simulink model "ExtendedKalmanFIlterRover"  (R2021a)
settings: Solver=VariableStepAuto  StartTime=0.0  StopTime=20.0  RelTol=1e-3
values from neighbouring files (symbols this model uses):
  Q = 1.2e-3    (= 0.0012)    [parameters.m]
  R = 5e-3    (= 0.005)    [parameters.m]
  Ts = 0.01    [parameters.m]
undefined symbols (not defined in the file or in its folder): K
libraries: robotlib x9, sharedTrackingLibrary x1
settings Model: Creator=user  LastModifiedBy=User
settings SolverCC: AlgebraicLoopSolver=TrustRegion
settings DebuggingCC: SFMachineParentedDataDiag=warning

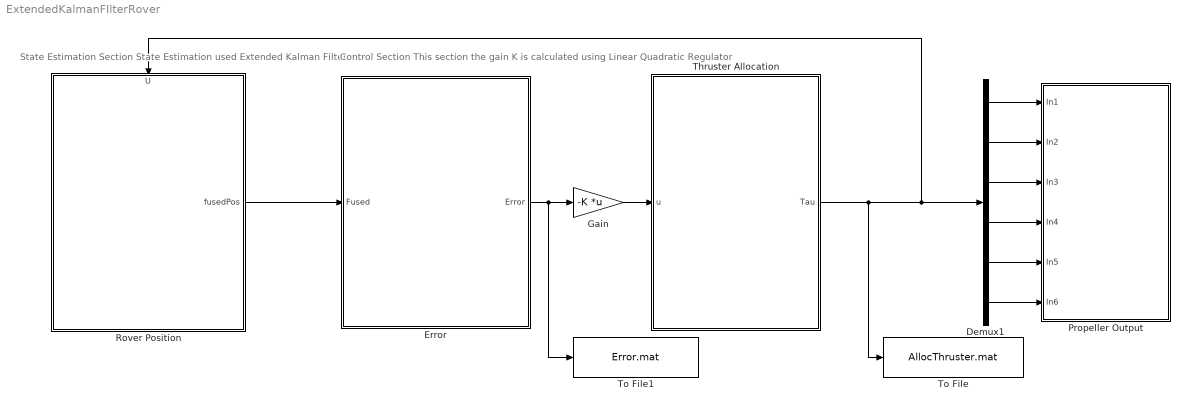
== system ExtendedKalmanFIlterRover ==
  note: State Estimation Section
      |
      | State Estimation used Extended Kalman Filter
  note: Control Section
      |
      | This section the gain K is calculated using Linear Quadratic Regulator
  Demux1 : Demux  Outputs=6
  Error : MATLAB Function  TreatAsAtomicUnit=on
  Gain : Gain  Gain=-K  Multiplication=Matrix(K*u)  RndMeth=Round
  Propeller Output : Subsystem
  Rover Position : Subsystem
      settings: PortSchema="{\"entries\":[{\"content\":{\"sides\":[{\"content\":{\"connectorIds\":[]},\"type\":\"ConnectorPlacement.EquallySpacedRectSide\",\"uuid\":\"70bf1008-d6b2-49b6-af88-753ab581769c\"},{\"content\":{\"connectorIds\":[\"Out1\"],\"side\":\"RIGHT\"},\"type\":\"ConnectorPlacement.EquallySpacedRectSide\",\"uuid\":\"04ddecda-8c46-4437-987b-fe54c22cd984\"},{\"content\":{\"connectorIds\":[\"In1\"],\"side\":\"TOP\"},\"type\":\"ConnectorPlacement.EquallySpacedRectSide\",\"uuid\":\"625a0b2a-12f2-4858-86ad-539843868268\"}]},\"type\":\"ConnectorPlacement.EquallySpacedConnector\",\"uuid\":\"e8b3dc5a-c0d9-4ca2-a6c5-b2c7be1821de\"}],\"packageUris\":[\"http://schema.mathworks.com/mf0/Connector/R2020b\"],\"version\":\"1.0\"}"
  Thruster Allocation : MATLAB Function  TreatAsAtomicUnit=on
  To File : ToFile  Filename=AllocThruster.mat  SaveFormat=Timeseries  SampleTime=Ts
  To File1 : ToFile  Filename=Error.mat  MatrixName=Error  SaveFormat=Timeseries  SampleTime=Ts
  wires:
  Thruster Allocation/1(Tau) -> To File/1, Demux1/1, Rover Position/1(U)
  Demux1/1 -> Propeller Output/1(In1)
  Demux1/2 -> Propeller Output/2(In2)
  Demux1/3 -> Propeller Output/3(In3)
  Demux1/4 -> Propeller Output/4(In4)
  Demux1/5 -> Propeller Output/5(In5)
  Demux1/6 -> Propeller Output/6(In6)
  Error/1(Error) -> To File1/1, Gain/1
  Rover Position/1(fusedPos) -> Error/1(Fused)
  Gain/1 -> Thruster Allocation/1(u)

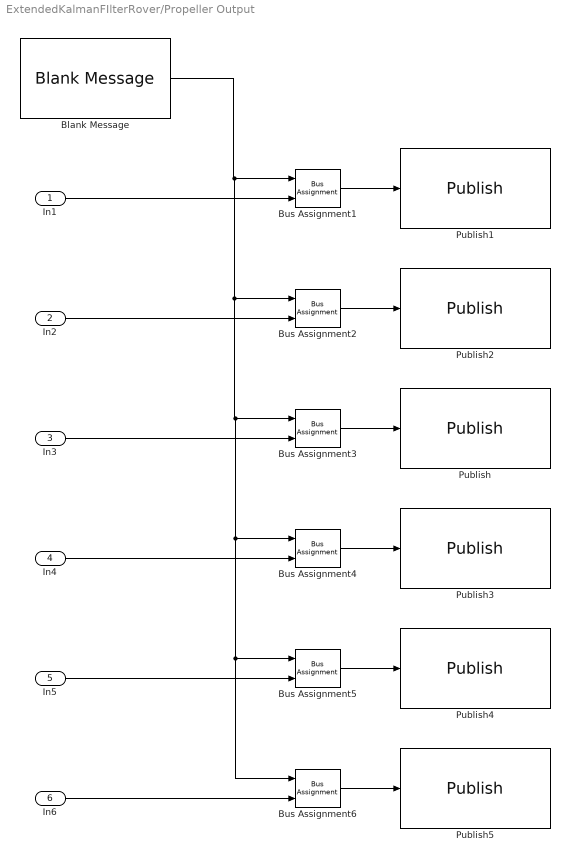
== system ExtendedKalmanFIlterRover/Propeller Output ==
  In1 : Inport
  In2 : Inport  Port=2
  In3 : Inport  Port=3
  In4 : Inport  Port=4
  In5 : Inport  Port=5
  In6 : Inport  Port=6
  Blank Message : robotlib/Blank Message  messageClass=Message  entityType=uuv_gazebo_ros_plugins_msgs/FloatStamped  messageType=uuv_gazebo_ros_plugins_msgs/FloatStamped  SampleTime=inf  legacyBusStruct=off
  Bus Assignment{1..6} (6 alike) : BusAssignment  AssignedSignals=Data
  Publish : robotlib/Publish  topicSource=Select from ROS network  topic=/bluerov2/thrusters/2/input  messageType=uuv_gazebo_ros_plugins_msgs/FloatStamped  legacyBusStruct=off  messageQueueLength=1
  Publish1 : robotlib/Publish  topicSource=Select from ROS network  topic=/bluerov2/thrusters/0/input  messageType=uuv_gazebo_ros_plugins_msgs/FloatStamped  legacyBusStruct=off  messageQueueLength=1
  Publish2 : robotlib/Publish  topicSource=Select from ROS network  topic=/bluerov2/thrusters/1/input  messageType=uuv_gazebo_ros_plugins_msgs/FloatStamped  legacyBusStruct=off  messageQueueLength=1
  Publish3 : robotlib/Publish  topicSource=Select from ROS network  topic=/bluerov2/thrusters/3/input  messageType=uuv_gazebo_ros_plugins_msgs/FloatStamped  legacyBusStruct=off  messageQueueLength=1
  Publish4 : robotlib/Publish  topicSource=Select from ROS network  topic=/bluerov2/thrusters/4/input  messageType=uuv_gazebo_ros_plugins_msgs/FloatStamped  legacyBusStruct=off  messageQueueLength=1
  Publish5 : robotlib/Publish  topicSource=Select from ROS network  topic=/bluerov2/thrusters/5/input  messageType=uuv_gazebo_ros_plugins_msgs/FloatStamped  legacyBusStruct=off  messageQueueLength=1
  wires:
  Bus Assignment5/1 -> Publish4/1
  Bus Assignment4/1 -> Publish3/1
  Bus Assignment3/1 -> Publish/1
  Bus Assignment2/1 -> Publish2/1
  Bus Assignment1/1 -> Publish1/1
  Bus Assignment6/1 -> Publish5/1
  Blank Message/1 -> Bus Assignment6/1, Bus Assignment5/1, Bus Assignment4/1, Bus Assignment3/1, Bus Assignment2/1, Bus Assignment1/1
  In1/1 -> Bus Assignment1/2
  In2/1 -> Bus Assignment2/2
  In3/1 -> Bus Assignment3/2
  In4/1 -> Bus Assignment4/2
  In5/1 -> Bus Assignment5/2
  In6/1 -> Bus Assignment6/2

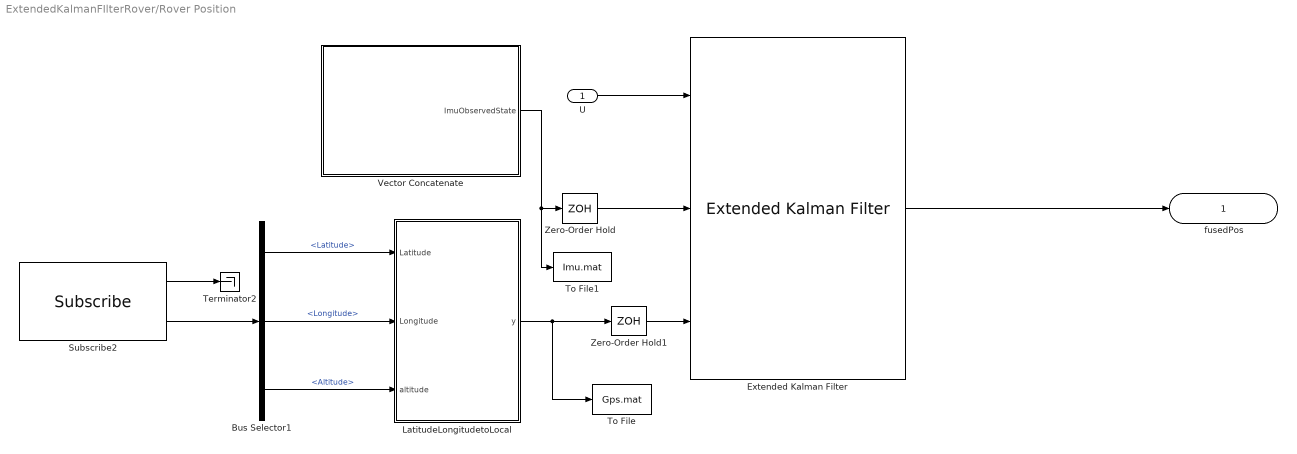
== system ExtendedKalmanFIlterRover/Rover Position ==
  U : Inport
  Bus Selector1 : BusSelector  OutputSignals=Latitude,Longitude,Altitude
  Extended Kalman Filter : sharedTrackingLibrary/Extended Kalman Filter  StateTransitionFcn=myStateTransitionFcn  HasStateTransitionJacobianFcn=off  HasAdditiveProcessNoise=Additive  ProcessNoise=diag([Q Q Q Q Q Q Q Q Q Q Q Q])  HasTimeVaryingProcessNoise=off  HasStateTransitionFcnExtraArgument=1  InitialState=[0 0 0 0 0 0 0 0 0 0 0 0]  InitialStateCovariance=1e-3  MeasurementFcn1=ImuMeasurementFcn  HasMeasurementJacobianFcn1=off  HasMeasurementEnablePort1=off  HasAdditiveMeasurementNoise1=Additive  MeasurementNoise1=diag([R R R R R R R R R R R R])  HasTimeVaryingMeasurementNoise1=off  HasMeasurementFcnExtraArgument1=0  MeasurementFcn2=GpsMeasurementFcn  HasMeasurementJacobianFcn2=off  HasMeasurementEnablePort2=off  HasAdditiveMeasurementNoise2=Additive  MeasurementNoise2=diag([R R R])  HasTimeVaryingMeasurementNoise2=off  HasMeasurementFcnExtraArgument2=0  MeasurementFcn3=myMeasurementFcn  HasMeasurementJacobianFcn3=off  HasMeasurementEnablePort3=off  HasAdditiveMeasurementNoise3=Additive  MeasurementNoise3=1  HasTimeVaryingMeasurementNoise3=off  HasMeasurementFcnExtraArgument3=0  MeasurementFcn4=myMeasurementFcn  HasMeasurementJacobianFcn4=off  HasMeasurementEnablePort4=off  HasAdditiveMeasurementNoise4=Additive  MeasurementNoise4=1  HasTimeVaryingMeasurementNoise4=off  HasMeasurementFcnExtraArgument4=0  MeasurementFcn5=myMeasurementFcn  HasMeasurementJacobianFcn5=off  HasMeasurementEnablePort5=off  HasAdditiveMeasurementNoise5=Additive  MeasurementNoise5=1  HasTimeVaryingMeasurementNoise5=off  HasMeasurementFcnExtraArgument5=0  EnableMultirate=off  StateTransitionFcnSampleTime=1  MeasurementFcn1SampleTime=1  MeasurementFcn2SampleTime=1  MeasurementFcn3SampleTime=1  MeasurementFcn4SampleTime=1  MeasurementFcn5SampleTime=1  UseCurrentEstimator=on  OutputStateCovariance=off  DataType=double  SampleTime=Ts  NumberOfMeasurements=2
      settings: SourceProductBaseCode=CT,DR,TF,ID,LP,NV,AR,RO,RR,UV,VE
  LatitudeLongitudetoLocal : MATLAB Function  TreatAsAtomicUnit=on
  Subscribe2 : robotlib/Subscribe  topicSource=Select from ROS network  topic=/bluerov2/gps  messageType=sensor_msgs/NavSatFix  SampleTime=Ts  legacyBusStruct=off  messageQueueLength=1
  Terminator2 : Terminator
  To File : ToFile  Filename=Gps.mat  MatrixName=Coordinate  SaveFormat=Timeseries  SampleTime=Ts
  To File1 : ToFile  Filename=Imu.mat  MatrixName=ImuCoordinate  SaveFormat=Timeseries  SampleTime=Ts
  Vector Concatenate : Subsystem
  Zero-Order Hold : ZeroOrderHold  SampleTime=-1
  Zero-Order Hold1 : ZeroOrderHold  SampleTime=-1
  fusedPos : Outport
  wires:
  Subscribe2/1 -> Terminator2/1
  Subscribe2/2 -> Bus Selector1/1
  Bus Selector1/1 -> LatitudeLongitudetoLocal/1(Latitude)  "<Latitude>"
  Bus Selector1/2 -> LatitudeLongitudetoLocal/2(Longitude)  "<Longitude>"
  Bus Selector1/3 -> LatitudeLongitudetoLocal/3(altitude)  "<Altitude>"
  Extended Kalman Filter/1 -> fusedPos/1
  Zero-Order Hold/1 -> Extended Kalman Filter/2
  Zero-Order Hold1/1 -> Extended Kalman Filter/3
  LatitudeLongitudetoLocal/1(y) -> To File/1, Zero-Order Hold1/1
  Vector Concatenate/1(ImuObservedState) -> To File1/1, Zero-Order Hold/1
  U/1 -> Extended Kalman Filter/1

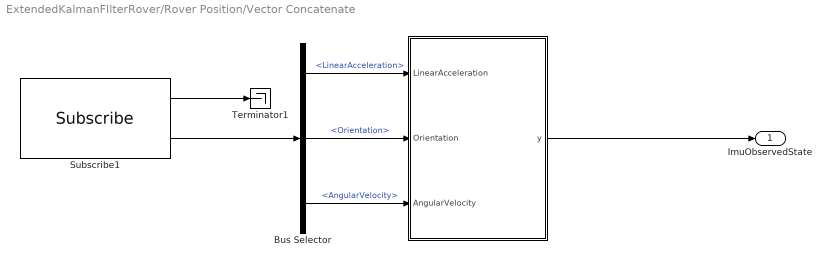
== system ExtendedKalmanFIlterRover/Rover Position/Vector Concatenate ==
  " " : MATLAB Function  TreatAsAtomicUnit=on
  Bus Selector : BusSelector  OutputSignals=LinearAcceleration,Orientation,AngularVelocity
  Subscribe1 : robotlib/Subscribe  topicSource=Specify your own  topic=/bluerov2/imu  messageType=sensor_msgs/Imu  SampleTime=Ts  legacyBusStruct=off  messageQueueLength=1
  Terminator1 : Terminator
  ImuObservedState : Outport
  wires:
  Subscribe1/1 -> Terminator1/1
  " "/1(y) -> ImuObservedState/1
  Subscribe1/2 -> Bus Selector/1
  Bus Selector/2 -> " "/2(Orientation)  "<Orientation>"
  Bus Selector/3 -> " "/3(AngularVelocity)  "<AngularVelocity>"
  Bus Selector/1 -> " "/1(LinearAcceleration)  "<LinearAcceleration>"

== matlab function ExtendedKalmanFIlterRover/Thruster Allocation ==
  data: u input; Tau output
function Tau = fcn(u)
Thruster_Configuration_Matrix = [0.707 0.707 -0.707 -0.707 0 0;0.707 -0.707 0.707 -0.707 0 0;0 0 0 0 1 1;0.051 -0.051 0.051 -0.051 -0.11 0.11;-0.051 -0.051 0.051 0.051 -0.0025 -0.0025;0.1655 -0.1655 -0.175 0.175 0 0];

% Tau = u;
Tau = pinv(u)*Thruster_Configuration_Matrix;

== matlab function ExtendedKalmanFIlterRover/Error ==
  data: Fused input; Error output
function Error = fcn(Fused)

%Set your reference
reference = [0;100;0;0;0;0;0;0;0;0;0;0];
Error = Fused - reference;

== matlab function ExtendedKalmanFIlterRover/Rover Position/Vector Concatenate/  ==
  data: LinearAcceleration input; Orientation input; y output; AngularVelocity input
function y = fcn(LinearAcceleration,Orientation,AngularVelocity)


VelocityX = cumtrapz(LinearAcceleration.X);
VelocityY = cumtrapz(LinearAcceleration.Y);
VelocityZ = cumtrapz(LinearAcceleration.Z);

PositionX = cumtrapz(VelocityX);
PositionY = cumtrapz(VelocityY);
PositionZ = cumtrapz(VelocityZ);


y = [PositionX;PositionY;PositionZ;Orientation.X;Orientation.Y;Orientation.Z;VelocityX;VelocityY;VelocityZ;AngularVelocity.X;AngularVelocity.Y;AngularVelocity.Z];

== matlab function ExtendedKalmanFIlterRover/Rover Position/LatitudeLongitudetoLocal ==
  data: Latitude input; y output; Longitude input; altitude input
function y = fcn(Latitude,Longitude,altitude)

origin = [-56.7189 -3.5156 0];

R = 6378137.0;  %relative to centre of the earth
OriginX = R*cos(deg2rad(origin(2)))*sin(deg2rad(origin(1)));
OriginY = R*sin(deg2rad(origin(2)))*sin(deg2rad(origin(1)));
OriginZ = R*cos(deg2rad(origin(1)));

StateR = 6378137.0 + altitude;  %relative to centre of the earth
StateX = StateR*cos(deg2rad(Longitude))*sin(deg2rad(Latitude));
StateY = StateR*sin(deg2rad(Longitude))*sin(deg2rad(Latitude));
StateZ = StateR*cos(deg2rad(Latitude));


y = [StateX-OriginX;StateY-OriginY;StateZ-OriginZ];
